simulink model "Ros_Actuator_Quadctor"  (R2022a)
settings: Solver=FixedStepAuto  StartTime=0.0  StopTime=inf  RelTol=1e-3  EnableMultiTasking=on
undefined symbols (not defined in the file): actuator, armed_time, command, control, onboard_control_sensors_enabled, onboard_control_sensors_present, param1, param2, system_id, target_system, timestamp, vehicle_type
libraries: ros2lib x10
settings Model: ExtModeTrigDuration=10  Creator=30258  LastModifiedBy=30258
settings SolverCC: PositivePriorityOrder=on
settings OptimizationCC: EnhancedBackFolding=on  PassReuseOutputArgsAs=Individual arguments  ZeroExternalMemoryAtStartup=off  ZeroInternalMemoryAtStartup=off  MaxStackSize=64  OptimizeBlockOrder=speed  DifferentSizesBufferReuse=on  OptimizationCustomize=off  EfficientTunableParamExpr=on
settings DebuggingCC: ParameterTunabilityLossMsg=error
settings HardwareCC: ProdBitPerPointer=32  ProdBitPerSizeT=32  ProdBitPerPtrDiffT=32  ProdLargestAtomicInteger=Long  ProdLargestAtomicFloat=Double  ProdWordSize=32  ProdLongLongMode=on  ProdHWDeviceType=ARM Compatible->ARM Cortex
settings SFSimCC: MATLABDynamicMemAlloc=off  SimTargetLang=C++
settings RTWCC: SystemTargetFile=ert.tlc  HardwareBoard=PX4 Pixhawk 4  TLCOptions="-aInlineSetEventsForThisBaseRateFcn=TLC_FALSE -aSuppressMultiTaskScheduler=TLC_FALSE  -aRateBasedStepFcn=0"  TemplateMakefile=ert_default_tmf  Toolchain=GNU Tools for PX4 Autopilots  TargetLang=C++
settings CodeAppCC: ForceParamTrailComments=on  IgnoreCustomStorageClasses=off  OperatorAnnotations=on  SimulinkDataObjDesc=on  SFDataObjDesc=on  InsertBlockDesc=on
settings ERTTargetCC: ExtModeTransport=3  ExtModeStaticAlloc=on  ExtModeStaticAllocSize=1024  ExtModeMexFile=ext_xcp  ExtModeIntrfLevel=Level2 - Open  RootIOFormat=Structure reference

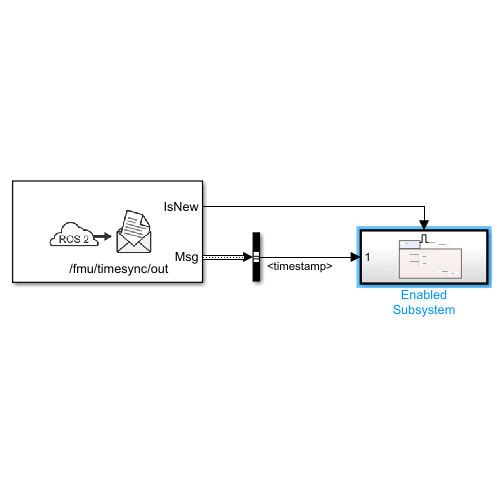
[thumbnail: Simulink's stored preview of the top-level diagram]
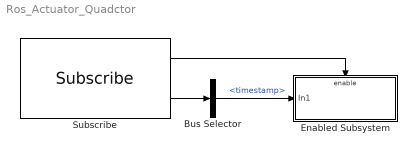
== system Ros_Actuator_Quadctor ==
  Bus Selector : BusSelector  OutputSignals=timestamp
  Enabled Subsystem : Subsystem  TreatAsAtomicUnit=on
  Subscribe : ros2lib/Subscribe  topicSource=Specify your own  topic=/fmu/timesync/out  messageType=px4_msgs/Timesync  sampleTime=-1  QOSHistory=Keep last  QOSDepth=1  QOSReliability=Reliable  QOSDurability=Volatile
      settings: SourceProductBaseCode=RR
  wires:
  Subscribe/1 -> Enabled Subsystem/Enable
  Subscribe/2 -> Bus Selector/1
  Bus Selector/1 -> Enabled Subsystem/1(In1)  "<timestamp>"

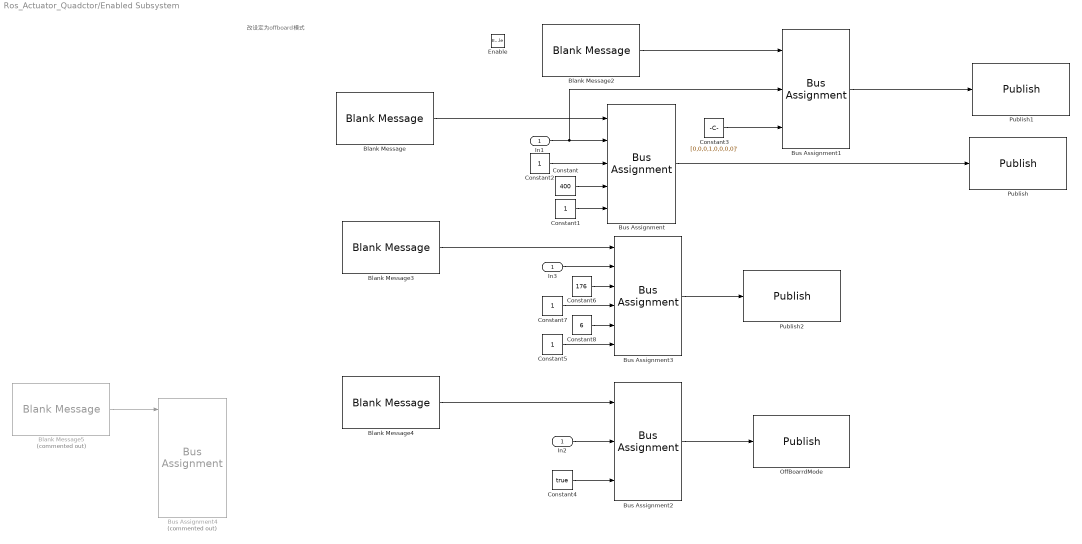
== system Ros_Actuator_Quadctor/Enabled Subsystem ==
  note: 改设定为offboard模式
  In1 : Inport
  Enable : EnablePort
  Blank Message : ros2lib/Blank Message  messageClass=Message  entityType=px4_msgs/VehicleCommand  messageType=px4_msgs/VehicleCommand  SampleTime=inf
      settings: SourceProductBaseCode=RR
  Blank Message2 : ros2lib/Blank Message  messageClass=Message  entityType=px4_msgs/ActuatorControls0  messageType=px4_msgs/ActuatorControls0  SampleTime=inf
      settings: SourceProductBaseCode=RR
  Blank Message3 : ros2lib/Blank Message  messageClass=Message  entityType=px4_msgs/VehicleCommand  messageType=px4_msgs/VehicleCommand  SampleTime=inf
      settings: SourceProductBaseCode=RR
  Blank Message4 : ros2lib/Blank Message  messageClass=Message  entityType=px4_msgs/OffboardControlMode  messageType=px4_msgs/OffboardControlMode  SampleTime=inf
      settings: SourceProductBaseCode=RR
  Blank Message5 : ros2lib/Blank Message  Commented=on  messageClass=Message  entityType=px4_msgs/VehicleStatus  messageType=px4_msgs/VehicleCommand  SampleTime=inf
      settings: SourceProductBaseCode=RR
  Bus Assignment : BusAssignment  AssignedSignals=timestamp,param1,command,target_system
  Bus Assignment1 : BusAssignment  AssignedSignals=timestamp,control
  Bus Assignment2 : BusAssignment  AssignedSignals=timestamp,actuator
  Bus Assignment3 : BusAssignment  AssignedSignals=timestamp,command,param1,param2,target_system
  Bus Assignment4 : BusAssignment  Commented=on  AssignedSignals=timestamp,onboard_control_sensors_enabled,vehicle_type,system_id,onboard_control_sensors_present,armed_time
  Constant : Constant  Value=400  OutDataTypeStr=uint32
  Constant1 : Constant  OutDataTypeStr=uint8
  Constant2 : Constant  OutDataTypeStr=single
  Constant3 : Constant  Value=[0,0,0,1,0,0,0,0]'  OutDataTypeStr=single
  Constant4 : Constant  Value=true  OutDataTypeStr=boolean
  Constant5 : Constant  OutDataTypeStr=uint8
  Constant6 : Constant  Value=176  VectorParams1D=off  OutDataTypeStr=uint32
  Constant7 : Constant  OutDataTypeStr=single
  Constant8 : Constant  Value=6  OutDataTypeStr=single
  In2 : InportShadow
  In3 : InportShadow
  OffBoarrdMode : ros2lib/Publish  topicSource=Specify your own  topic=/fmu/offboard_control_mode/in  messageType=px4_msgs/OffboardControlMode  QOSHistory=Keep last  QOSDepth=1  QOSReliability=Reliable  QOSDurability=Volatile
      settings: SourceProductBaseCode=RR
  Publish : ros2lib/Publish  topicSource=Specify your own  topic=/fmu/vehicle_command/in  messageType=px4_msgs/VehicleCommand  QOSHistory=Keep last  QOSDepth=1  QOSReliability=Reliable  QOSDurability=Volatile
      settings: SourceProductBaseCode=RR
  Publish1 : ros2lib/Publish  topicSource=Specify your own  topic=/fmu/actuator_controls0/in  messageType=px4_msgs/ActuatorControls0  QOSHistory=Keep last  QOSDepth=1  QOSReliability=Reliable  QOSDurability=Volatile
      settings: SourceProductBaseCode=RR
  Publish2 : ros2lib/Publish  topicSource=Specify your own  topic=/fmu/vehicle_command/in  messageType=px4_msgs/VehicleCommand  QOSHistory=Keep last  QOSDepth=1  QOSReliability=Reliable  QOSDurability=Volatile
      settings: SourceProductBaseCode=RR
  wires:
  Blank Message/1 -> Bus Assignment/1
  Constant/1 -> Bus Assignment/4
  In1/1 -> Bus Assignment/2, Bus Assignment1/2
  Constant1/1 -> Bus Assignment/5
  Constant2/1 -> Bus Assignment/3
  Bus Assignment/1 -> Publish/1
  Bus Assignment1/1 -> Publish1/1
  Blank Message2/1 -> Bus Assignment1/1
  Blank Message4/1 -> Bus Assignment2/1
  Bus Assignment2/1 -> OffBoarrdMode/1
  In2/1 -> Bus Assignment2/2
  Constant4/1 -> Bus Assignment2/3
  Bus Assignment3/1 -> Publish2/1
  Blank Message3/1 -> Bus Assignment3/1
  Constant5/1 -> Bus Assignment3/6
  Constant8/1 -> Bus Assignment3/5
  Blank Message5/1 -> Bus Assignment4/1
  In3/1 -> Bus Assignment3/2
  Constant6/1 -> Bus Assignment3/3
  Constant7/1 -> Bus Assignment3/4
  Constant3/1 -> Bus Assignment1/3
